simulink model "Balancing_Logic"  (R2024b)
settings: configuration reference "BMS_Sw_CodeGenConfig" (kept outside this file)
undefined symbols (not defined in the file): BalNotActWait, BalOffWait, BalOnWait, flgEnBalancing, Ns_Module, NumModules, TargetDeltaV
settings Model: DataDictionary=DD_Balancing_Logic.sldd  ExtModeTrigDuration=5  Creator=cpatel  LastModifiedBy=18811
settings ConfigSetRef: SourceName=BMS_Sw_CodeGenConfig

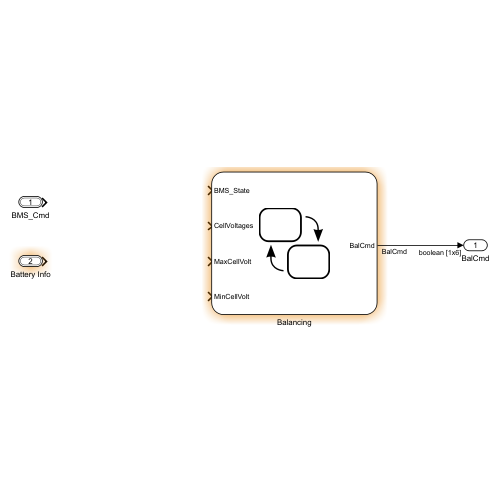
[thumbnail: Simulink's stored preview of the top-level diagram]
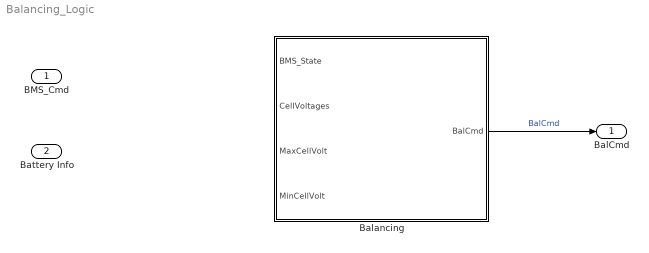
== system Balancing_Logic ==
  BMS_Cmd : Inport  OutDataTypeStr=Bus: BMS_Cmd
  Battery Info : Inport  Port=2  OutDataTypeStr=Bus: Battery_Info
  Balancing : Stateflow chart  TreatAsAtomicUnit=on  VariantControl=(default)
  BalCmd : Outport  OutDataTypeStr=boolean  PortDimensions=[1,NumModules*Ns_Module]  SampleTime=[5,0]  VectorParamsAs1DForOutWhenUnconnected=off
  wires:
  Balancing/1(BalCmd) -> BalCmd/1  "BalCmd"

== stateflow chart Balancing_Logic/Balancing ==
  state BalancingOFF
    en:
    BalCmd(:,:) = false;
    en,du:
    DeltaCellVolt = MaxCellVolt - MinCellVolt;
  state BalancingON
    en, du:
    DeltaCellVolt = MaxCellVolt - MinCellVolt;
    state BalActive
      en, du:
      BalCmd = ((CellVoltages - MinCellVolt) > TargetDeltaV/2)';
      flgBalCompl = all(~BalCmd);
    state BalNotActive
    (default) -> BalActive
    BalNotActive -> BalActive [order 1] : [after(BalNotActWait,sec) && ...
        | DeltaCellVolt > TargetDeltaV]
    BalActive -> BalNotActive : [flgBalCompl]
  (default) -> BalancingOFF : {flgBalCompl = true;}
  BalancingOFF -> BalancingON : [flgEnBalancing && ...
      | BMS_State ~= BMS_State_Enum.BMS_Driving && ...
      | after(BalOffWait,sec) && ...
      | DeltaCellVolt > TargetDeltaV]
  BalancingON -> BalancingOFF : [BMS_State == BMS_State_Enum.BMS_Driving] %In Driving State
  BalNotActive -> BalancingOFF [order 2] : [after(BalOnWait,sec)]
  data: BMS_State input Enum: BMS_State_Enum; CellVoltages input single; TargetDeltaV parameter; BalCmd output boolean size=[1,Ns_Module*NumModules] =boolean(zeros(1,Ns_Module*NumModules)); flgBalCompl local; MaxCellVolt input single; MinCellVolt input single; BalNotActWait parameter; BalOffWait parameter; BalOnWait parameter; flgEnBalancing parameter; DeltaCellVolt local single =single(0)
